simulink model "ukol_8_model"  (R2017a)
settings: Solver=VariableStepAuto  StartTime=0.0  StopTime=10.0  MaxStep=1e-3  RelTol=1e-3  EnableMultiTasking=on
values from neighbouring files (symbols this model uses):
  A = [0 1; -1.44 -0.36]    [ukol_5_script.m]
  B = [0; 1]    [ukol_5_script.m]
  C = [7.2 0; 0 7.2]    [ukol_5_script.m]    (also in ukol_8_script.m = C_1; ukol_9_script.m)
  L = [0.505555; 0.173555]    [ukol_8_script.m]
settings Model: Creator=kuhaj  LastModifiedBy=tomas
settings DataIOCC: LimitDataPoints=on
settings OptimizationCC: LifeSpan=inf
settings DebuggingCC: AllowSymbolicDim=off  SFUnexpectedBacktrackingDiag=warning  SFNoUnconditionalDefaultTransitionDiag=warning  SFExecutionAtInitializationDiag=none
settings ModelReferenceCC: PropagateSignalLabelsOutOfModel=off
settings GRTTargetCC: TargetLangStandard=C89/C90 (ANSI)
settings ConfigComp: CovMetricSettings=dw  CovHtmlReporting=on  CovSaveCumulativeToWorkspaceVar=on  CovSaveSingleToWorkspaceVar=on  CovExternalEMLEnable=off

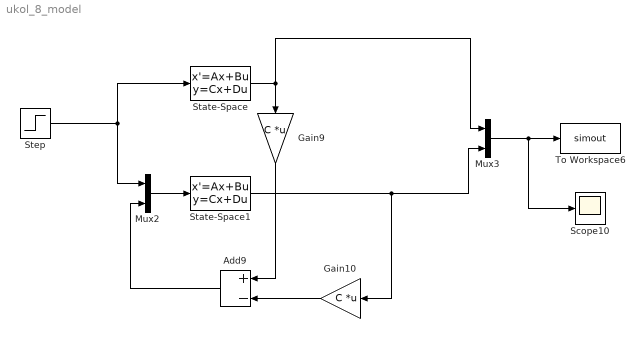
== system ukol_8_model ==
  Add9 : Sum  Inputs=+-
  Gain10 : Gain  Gain=C  Multiplication=Matrix(K*u)
  Gain9 : Gain  Gain=C  Multiplication=Matrix(K*u)
  Mux2 : Mux  Inputs=2
  Mux3 : Mux  Inputs=2
  Scope10 : Scope
  State-Space : StateSpace  A=A  B=B  C=eye(2)  D=[0 ;0]  X0=[2; -1]
  State-Space1 : StateSpace  A=A  B=[B L]  C=eye(2)  D=zeros(2)  X0=[-2;1]
  Step : Step  SampleTime=0
  To Workspace6 : ToWorkspace  VariableName=simout  SaveFormat=Timeseries  SampleTime=-1
  wires:
  Mux2/1 -> State-Space1/1
  Mux3/1 -> To Workspace6/1, Scope10/1
  State-Space/1 -> Mux3/1, Gain9/1
  Gain9/1 -> Add9/1
  State-Space1/1 -> Mux3/2, Gain10/1
  Gain10/1 -> Add9/2
  Add9/1 -> Mux2/2
  Step/1 -> Mux2/1, State-Space/1
